simulink model "SimParking"  (R2017b)
settings: Solver=VariableStepAuto  StartTime=0.0  StopTime=1761  RelTol=1e-3
libraries: neural x1111
(part 60 of 60)

== system SimParking/NARX Neural Network/Layer 4/Delays 1 ==
  "p{4}" : Inport  PortDimensions=50  SampleTime=1
      mask Display: e = 0.06;c1 = [120 230 180]/255;c2 = ([120 230 180]+0)/(256+128);c3 = ([120 230 180]+128)/(256+128);patch([0 1 1 0],[0 0 1 1],c1);patch([0 1 1 1-e 1-e 0+e],[0 0 1 1-e 0+e 0+e],c2);patch([0 0 1 1-e 0+e 0+e],[0 1 1 1-e 1-e 0+e],c3);plot([0 1 1 0 0],[0 0 1 1 0]);
  mux : Mux  Inputs=1
      mask Display: e = 0.06;c1 = [120 150 230]/255;c2 = ([120 150 230]+0)/383;c3 = ([120 150 230]+128)/383;patch([0 1 1 0],[0 0 1 1],c1);patch([0 1 1 1-e 1-e 0+e],[0 0 1 1-e 0+e 0+e],c2);patch([0 0 1 1-e 0+e 0+e],[0 1 1 1-e 1-e 0+e],c3);plot([0 1 1 0 0],[0 0 1 1 0]);disp('Mux')
  "pd{4,3}" : Outport
      mask Display: e = 0.06;c1 = [120 230 180]/255;c2 = ([120 230 180]+0)/(256+128);c3 = ([120 230 180]+128)/(256+128);patch([0 1 1 0],[0 0 1 1],c1);patch([0 1 1 1-e 1-e 0+e],[0 0 1 1-e 0+e 0+e],c2);patch([0 0 1 1-e 0+e 0+e],[0 1 1 1-e 1-e 0+e],c3);plot([0 1 1 0 0],[0 0 1 1 0]);
  wires:
  "p{4}"/1 -> mux/1
  mux/1 -> "pd{4,3}"/1

== system SimParking/NARX Neural Network/Layer 4/LW{4,3} ==
  "ad{4,3}" : Inport  PortDimensions=50  SampleTime=1
      mask Display: e = 0.06;c1 = [120 230 180]/255;c2 = ([120 230 180]+0)/(256+128);c3 = ([120 230 180]+128)/(256+128);patch([0 1 1 0],[0 0 1 1],c1);patch([0 1 1 1-e 1-e 0+e],[0 0 1 1-e 0+e 0+e],c2);patch([0 0 1 1-e 0+e 0+e],[0 1 1 1-e 1-e 0+e],c3);plot([0 1 1 0 0],[0 0 1 1 0]);
  "IW{4,3}(1,:)'" : Constant  Value=[-0.442215178662435814960218749547493644058704376220703125;0.506766820979722698581326767452992498874664306640625;-0.86703428073242283513621941892779432237148284912109375;0.11376943079587820140119447387405671179294586181640625;-0.71889426329957795136493814425193704664707183837890625;-0.09974344392070545739503728555064299143850803375244140625;0.3759851980110682223568119297851808369159698486328125;-0.666899170430979904011792314122430980205535888671875;-0.8991315320430317559186050857533700764179229736328125;-0.214448889970179024100360720694880001246929168701171875;0.238464166115718467775508315753540955483913421630859375;0.03635998124373072959425456929238862358033657073974609375;0.1054218745135833135151415262953378260135650634765625;-0.379054030355621296433099587375181727111339569091796875;-0.54307240161429082281330238402006216347217559814453125;-0.340390583232753118902991218419629149138927459716796875;0.055696823664790000296687111358551192097365856170654296875;-0.64702803741724401742629879663581959903240203857421875;0.716367455798579744197240870562382042407989501953125;0.688097259530895843937514655408449470996856689453125;0.002271387091319964322833069303442243835888803005218505859375;0.06149809470614812922928393845722894184291362762451171875;-0.72106529313895684207835756751592271029949188232421875;0.0627496918121341895613340966519899666309356689453125;-0.2387491576988605423981226749674533493816852569580078125;-0.256911752380252045302455599085078574717044830322265625;0.1845396851944771932085842536253039725124835968017578125;0.032054190633197886250993491330518736504018306732177734375;-0.334234043048197870806603759774588979780673980712890625;-0.0445664696228165457814185401730355806648731231689453125;0.20328975479023991823623873642645776271820068359375;-0.5965977405993025950436958737554959952831268310546875;-0.073179443675099598021205338227446191012859344482421875;0.349882572653665346873452790532610379159450531005859375;0.6666711472660804549406066144001670181751251220703125;-0.0798729737614377877097382452120655216276645660400390625;0.334596484217011547190878673063707537949085235595703125;-0.2621555285105845456428141915239393711090087890625;0.0574467082444672094698745468122069723904132843017578125;-0.2629373653338198391082869420642964541912078857421875;-0.183747854966513968211216933923424221575260162353515625;0.69891957708506680102544805777142755687236785888671875;-0.58954369996475097792654196382500231266021728515625;0.08744619396181975423676391301341936923563480377197265625;0.62637247011491747894496029402944259345531463623046875;-0.03341383902310122999690378264858736656606197357177734375;-0.1414442596372735838627932025701738893985748291015625;0.08544925584923381001178910310045466758310794830322265625;0.08239371069819294290947908621092210523784160614013671875;-0.89106382613495715983020772910094819962978363037109375]
      mask Display: e = 0.06;c1 = [120 150 230]/255;c2 = ([120 150 230]+0)/383;c3 = ([120 150 230]+128)/383;patch([0 1 1 0],[0 0 1 1],c1);patch([0 1 1 1-e 1-e 0+e],[0 0 1 1-e 0+e 0+e],c2);patch([0 0 1 1-e 0+e 0+e],[0 1 1 1-e 1-e 0+e],c3);plot([0 1 1 0 0],[0 0 1 1 0]);disp('weights');
  "IW{4,3}(2,:)'" : Constant  Value=[0.9538547442894778072286499082110822200775146484375;-0.0207426311995310037883388787349758786149322986602783203125;0.10205658934457302600140593540345435030758380889892578125;-0.593567824973260993459689416340552270412445068359375;0.3678525783666388715431594391702674329280853271484375;-0.87068575530929293027071480537415482103824615478515625;0.275190347008952118645908058169879950582981109619140625;-0.50592625774160848717286853570840321481227874755859375;0.441700755854442184134001081474707461893558502197265625;0.94616788833147025261638418669463135302066802978515625;0.30287268042630766107237150208675302565097808837890625;-0.90706914271350658207637707164394669234752655029296875;-0.048156245389165248937946017804279108531773090362548828125;-0.137313653823402492815120012892293743789196014404296875;-0.048848303488187062859626763611231581307947635650634765625;-1.0045739770435193616293645391124300658702850341796875;-0.809766426224302282577127698459662497043609619140625;0.6707627739718129422641368364566005766391754150390625;-0.0927408534346988722152360651307390071451663970947265625;0.84607464021382394747661237488500773906707763671875;0.07387655021692578205527723866907763294875621795654296875;0.71812695012863592136653778652544133365154266357421875;0.94863528836543176137041655238135717809200286865234375;0.037460683788145550388026805421759490855038166046142578125;-0.3793847882533487592127130483277142047882080078125;0.250241465401251750311217847411171533167362213134765625;-0.47183869232020969608498717207112349569797515869140625;-0.1684550145735861093054808179658721201121807098388671875;-0.43833244069577237400636704478529281914234161376953125;-0.1544250183683676114210214791455655358731746673583984375;-0.341488093502938683254654961274354718625545501708984375;-0.20463305366874695589984867183375172317028045654296875;-0.09846900788082786626365106030789320357143878936767578125;0.217478508965465999747124214991345070302486419677734375;0.53715565600236148124935198211460374295711517333984375;-0.6184073682752295741948955765110440552234649658203125;-0.352510865886858704154604993163957260549068450927734375;0.30161062061757182295451684694853611290454864501953125;-0.29825016786288693904083402230753563344478607177734375;-0.63770366049029636457134984084405004978179931640625;-0.169978598776351130794637356302700936794281005859375;0.3542355391815823484336078763590194284915924072265625;0.0846570453521134635987976935211918316781520843505859375;0.2466714622857260341692864358265069313347339630126953125;0.431815915068420708156082810091902501881122589111328125;-0.6318370953653269506133938193670473992824554443359375;0.381253186810359689928873194730840623378753662109375;-0.7350004593227079663364520456525497138500213623046875;-0.88171718362602968799279778977506794035434722900390625;-0.34586500973419209703507704034564085304737091064453125]
      mask Display: e = 0.06;c1 = [120 150 230]/255;c2 = ([120 150 230]+0)/383;c3 = ([120 150 230]+128)/383;patch([0 1 1 0],[0 0 1 1],c1);patch([0 1 1 1-e 1-e 0+e],[0 0 1 1-e 0+e 0+e],c2);patch([0 0 1 1-e 0+e 0+e],[0 1 1 1-e 1-e 0+e],c3);plot([0 1 1 0 0],[0 0 1 1 0]);disp('weights');
  "IW{4,3}(3,:)'" : Constant  Value=[-0.79895068745796760101285372002166695892810821533203125;0.813214202878986380795822697109542787075042724609375;0.309560726098363658831402744908700697124004364013671875;0.801277884380084959303758296300657093524932861328125;-0.81982255746120202832827317251940257847309112548828125;-0.290152388940309979847853583123651333153247833251953125;0.61580497962002256340241501675336621701717376708984375;-0.01355301459405609983133178531033991021104156970977783203125;0.317235039214918856931291202272404916584491729736328125;-0.089632364254139673676036181859672069549560546875;0.01337233247231379464070588625190794118680059909820556640625;0.1761743515632348822119723763535148464143276214599609375;-0.00645596423721033103870770020193958771415054798126220703125;0.4664348535908329207444467101595364511013031005859375;-0.01502401148158654352327001646472126594744622707366943359375;0.0194473748661927285652506469659783761017024517059326171875;-0.50425579722880120581152141312486492097377777099609375;-0.1799526213645722128031678721526986919343471527099609375;-0.10960163707921651010668284698112984187901020050048828125;0.1149599967537522082761114461391116492450237274169921875;0.0015926399123151091692662806309499501367099583148956298828125;-0.171292650124957479551568440001574344933032989501953125;0.70081764907341492776282620980055071413516998291015625;-1.1653163865211755290118844641256146132946014404296875;-0.0155430099580947077286818824859437881968915462493896484375;-0.879821554124404325847308427910320460796356201171875;0.003027292391034380227010647246288499445654451847076416015625;-0.1893603425842843301918350107371225021779537200927734375;-0.4805693038291958263386050020926631987094879150390625;0.0506283247169976580170924762569484300911426544189453125;-0.0025786081990634558518127317228163519757799804210662841796875;-0.18978778134950158307248102573794312775135040283203125;0.98042371873249500868752193127875216305255889892578125;-0.01088290305263289216297639683261877507902681827545166015625;-0.36434696020782364467294200949254445731639862060546875;-0.51265073350046075351116314777755178511142730712890625;0.1479028497553919463403104828103096224367618560791015625;0.00877379380860734796321320771994578535668551921844482421875;0.00291646313697101720874282904105712077580392360687255859375;0.3280109221698068733275022168527357280254364013671875;-0.092365159295790866256226081532076932489871978759765625;0.8289327170572835523643107080715708434581756591796875;-0.58788671594000307951688455432304181158542633056640625;0.330148913366270002622826496008201502263545989990234375;0.24101462180813804092593954919720999896526336669921875;0.562625228125702481207781602279283106327056884765625;-0.437992490356455321798279101130901835858821868896484375;0.443375442682015064033151929834275506436824798583984375;0.62744540881162913503743538967682980000972747802734375;-0.66498878069126143852685117963119409978389739990234375]
      mask Display: e = 0.06;c1 = [120 150 230]/255;c2 = ([120 150 230]+0)/383;c3 = ([120 150 230]+128)/383;patch([0 1 1 0],[0 0 1 1],c1);patch([0 1 1 1-e 1-e 0+e],[0 0 1 1-e 0+e 0+e],c2);patch([0 0 1 1-e 0+e 0+e],[0 1 1 1-e 1-e 0+e],c3);plot([0 1 1 0 0],[0 0 1 1 0]);disp('weights');
  Mux : Mux  Inputs=3
      mask Display: e = 0.06;c1 = [120 150 230]/255;c2 = ([120 150 230]+0)/383;c3 = ([120 150 230]+128)/383;patch([0 1 1 0],[0 0 1 1],c1);patch([0 1 1 1-e 1-e 0+e],[0 0 1 1-e 0+e 0+e],c2);patch([0 0 1 1-e 0+e 0+e],[0 1 1 1-e 1-e 0+e],c3);plot([0 1 1 0 0],[0 0 1 1 0]);disp('Mux');
  dotprod1 : neural/Weight Functions/dotprod
  dotprod2 : neural/Weight Functions/dotprod
  dotprod3 : neural/Weight Functions/dotprod
  "lz{4,3}" : Outport
      mask Display: e = 0.06;c1 = [120 230 180]/255;c2 = ([120 230 180]+0)/(256+128);c3 = ([120 230 180]+128)/(256+128);patch([0 1 1 0],[0 0 1 1],c1);patch([0 1 1 1-e 1-e 0+e],[0 0 1 1-e 0+e 0+e],c2);patch([0 0 1 1-e 0+e 0+e],[0 1 1 1-e 1-e 0+e],c3);plot([0 1 1 0 0],[0 0 1 1 0]);
  wires:
  "IW{4,3}(1,:)'"/1 -> dotprod1/1
  "ad{4,3}"/1 -> dotprod1/2, dotprod2/2, dotprod3/2
  dotprod1/1 -> Mux/1
  "IW{4,3}(2,:)'"/1 -> dotprod2/1
  dotprod2/1 -> Mux/2
  "IW{4,3}(3,:)'"/1 -> dotprod3/1
  dotprod3/1 -> Mux/3
  Mux/1 -> "lz{4,3}"/1
